simulink model "distributed_UIO_4nodes_directed"  (R2023a)
settings: Solver=VariableStepAuto  StartTime=0.0  StopTime=10  FixedStep=1e-6  RelTol=1e-6
values from neighbouring files (symbols this model uses):
  A = [-1   0    0   0   0   0 ... (first row only)    [init_simulink_DO.m]    (also in main.m)
  Adj = aij    [init_simulink_DO.m]
  gamma = 219.7065    [init_simulink_DO.m]    (also in main.m)
  H1 = [  1 0 0 2 0 0 ... (first row only)    [init_simulink_DO.m]    (also in main.m)
  H2 = [2 0 1 0 0 1]    [init_simulink_DO.m]    (also in main.m)
  H3 = [0 0 0 2 0 0]    [init_simulink_DO.m]    (also in main.m)
  H4 = [1 0 2 0 0 0 ... (first row only)    [init_simulink_DO.m]    (also in main.m)
  L1 = [0.1661 0.1661 ... (first row only)    [init_simulink_DO.m]    (also in main.m)
  L2 = [3.5770 ... (first row only)    [init_simulink_DO.m]    (also in main.m)
  L3 = [0 ... (first row only)    [init_simulink_DO.m]    (also in main.m)
  L4 = [-2.2551    0.3970 ... (first row only)    [init_simulink_DO.m]    (also in main.m)
  M1 = [0.0037    0       0   0       0   0 ... (first row only)    [init_simulink_DO.m]    (also in main.m)
  M2 = [0.0512     0.0879      -0.1315     -0.1416     -0.0429     0.0297 ... (first row only)    [init_simulink_DO.m]    (also in main.m)
  M3 = [1  0   0   0       0   0 ... (first row only)    [init_simulink_DO.m]    (also in main.m)
  M4 = [0.0390     0.0293      -0.0195     -0.1186     -0.1410     0.0409 ... (first row only)    [init_simulink_DO.m]    (also in main.m)
  x0 = [1, 3, -2, -3, -1, 2]'    [init_simulink_DO.m]
settings Model: Creator=gy116  LastModifiedBy=Quang Huy Nugyen
settings SolverCC: AlgebraicLoopSolver=LineSearch
settings DataIOCC: ReturnWorkspaceOutputs=off
settings DebuggingCC: UnconnectedInputMsg=warning  UnconnectedOutputMsg=warning  UnconnectedLineMsg=warning  ArithmeticOperatorsInVariantConditions=warning
settings ModelReferenceCC: EnableRefExpFcnMdlSchedulingChecks=on
settings SFSimCC: SimUseLocalCustomCode=off  CustomCodeUndefinedFunction=UseInterfaceOnly
settings RTWCC: RTWUseLocalCustomCode=off  DLArmComputeVersion=19.05
settings CodeAppCC: StateflowObjectComments=on

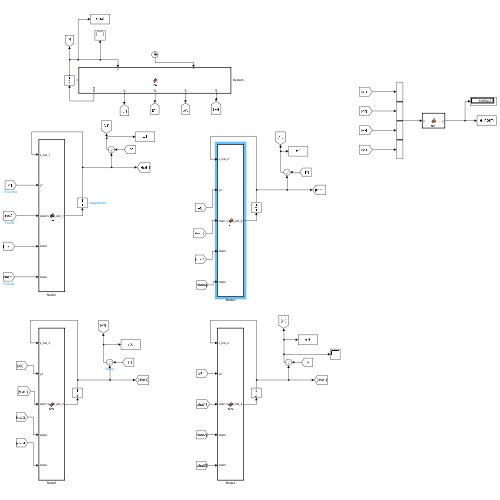
[thumbnail: Simulink's stored preview of the top-level diagram]
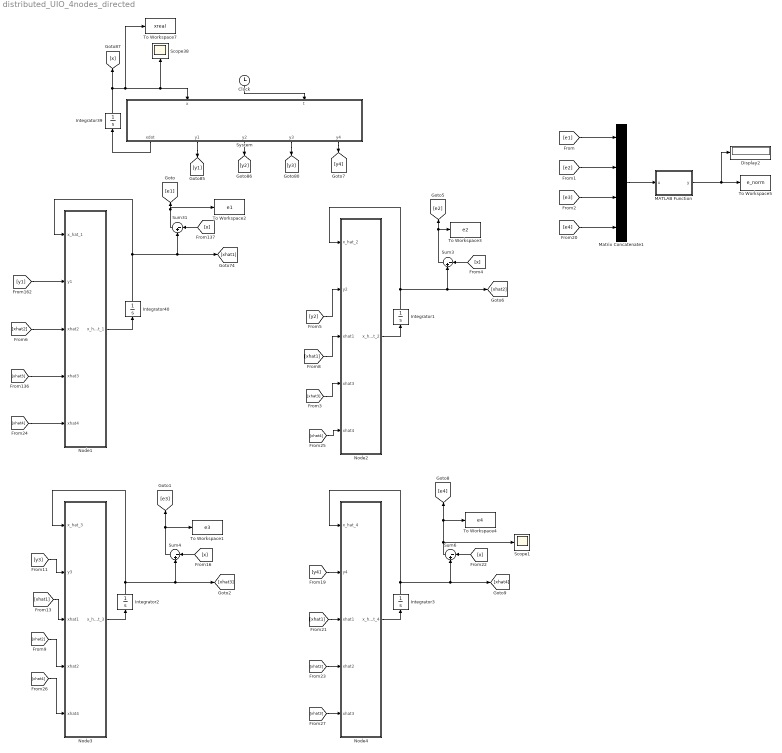
== system distributed_UIO_4nodes_directed ==
  Clock : Clock
  Display2 : Display
  Integrator{1..3,40} (4 alike) : Integrator  InitialCondition=0*x0
  Integrator39 : Integrator  InitialCondition=x0
  MATLAB Function : MATLAB Function  TreatAsAtomicUnit=on
  Matrix Concatenate1 : Concatenate  NumInputs=4  ConcatenateDimension=2
  Node1 : MATLAB Function  TreatAsAtomicUnit=on
  Node2 : MATLAB Function  TreatAsAtomicUnit=on
  Node3 : MATLAB Function  TreatAsAtomicUnit=on
  Node4 : MATLAB Function  TreatAsAtomicUnit=on
  Scope1 : Scope
  Scope38 : Scope
  Sum{3..4,6,31} (4 alike) : Sum  Inputs=|-+
  System : MATLAB Function  TreatAsAtomicUnit=on
  To Workspace1 : ToWorkspace  VariableName=e3  SaveFormat=Structure With Time  SampleTime=-1
  To Workspace2 : ToWorkspace  VariableName=e1  SaveFormat=Structure With Time  SampleTime=-1
  To Workspace3 : ToWorkspace  VariableName=e2  SaveFormat=Structure With Time  SampleTime=-1
  To Workspace4 : ToWorkspace  VariableName=e4  SaveFormat=Structure With Time  SampleTime=-1
  To Workspace5 : ToWorkspace  VariableName=e_norm  SaveFormat=Structure With Time  SampleTime=-1
  To Workspace7 : ToWorkspace  VariableName=xreal  SaveFormat=Structure With Time  SampleTime=-1
  wires:
  [e1] -> Matrix Concatenate1/1
  [e2] -> Matrix Concatenate1/2
  [e3] -> Matrix Concatenate1/3
  [e4] -> Matrix Concatenate1/4
  [x] -> Sum6/1
  [xhat1] -> Node3/3(xhat1)
  Sum6/1 -> Scope1/1, To Workspace4/1, [e4]
  Node1/1(x_hat_dot_1) -> Integrator40/1
  [y1] -> Node1/2(y1)
  Integrator2/1 -> Sum4/2, [xhat3], Node3/1(x_hat_3)
  Integrator40/1 -> Sum31/2, [xhat1], Node1/1(x_hat_1)
  Node4/1(x_hat_dot_4) -> Integrator3/1
  Integrator39/1 -> To Workspace7/1, System/1(x), Scope38/1, [x]
  Integrator1/1 -> Sum3/2, [xhat2], Node2/1(x_hat_2)
  [xhat4] -> Node2/5(xhat4)
  System/5(y4) -> [y4]
  System/2(y1) -> [y1]
  [y4] -> Node4/2(y4)
  [xhat2] -> Node4/4(xhat2)
  [xhat3] -> Node4/5(xhat3)
  Sum3/1 -> To Workspace3/1, [e2]
  System/1(xdot) -> Integrator39/1
  Clock/1 -> System/2(t)
  [xhat2] -> Node1/3(xhat2)
  System/4(y3) -> [y3]
  [x] -> Sum31/1
  [xhat4] -> Node3/5(xhat4)
  [y2] -> Node2/2(y2)
  [y3] -> Node3/2(y3)
  Sum31/1 -> To Workspace2/1, [e1]
  [xhat3] -> Node2/4(xhat3)
  [xhat2] -> Node3/4(xhat2)
  System/3(y2) -> [y2]
  [xhat3] -> Node1/4(xhat3)
  [x] -> Sum3/1
  Node2/1(x_hat_dot_2) -> Integrator1/1
  Node3/1(x_hat_dot_3) -> Integrator2/1
  [x] -> Sum4/1
  [xhat1] -> Node2/3(xhat1)
  Sum4/1 -> To Workspace1/1, [e3]
  Integrator3/1 -> Sum6/2, [xhat4], Node4/1(x_hat_4)
  [xhat1] -> Node4/3(xhat1)
  [xhat4] -> Node1/5(xhat4)
  Matrix Concatenate1/1 -> MATLAB Function/1(u)
  MATLAB Function/1(y) -> Display2/1, To Workspace5/1

== matlab function distributed_UIO_4nodes_directed/System ==
  data: x input; t input; A parameter; xdot output; y1 output; y2 output; y3 output; H2 parameter; H3 parameter; H1 parameter; H4 parameter; y4 output
function [xdot,y1,y2,y3,y4] = fcn(x,t,A,H2, H3, H1, H4)
xdot = A*x ;


y1 = H1*x;
y2 = H2*x;
y3 = H3*x;
y4 = H4*x;

== matlab function distributed_UIO_4nodes_directed/Node2 ==
  data: x_hat_2 input; y2 input; xhat1 input; xhat3 input; xhat4 input; x_hat_dot_2 output; L2 parameter; gamma parameter; Adj parameter; H2 parameter; A parameter; M2 parameter
function x_hat_dot_2   = fcn(x_hat_2,y2,xhat1,xhat3,xhat4,L2, gamma, Adj, H2, A, M2)

commu2 =  Adj(2,1)*(xhat1-x_hat_2) + Adj(2,3)*(xhat3-x_hat_2) + Adj(2,4)*(xhat4-x_hat_2);

x_hat_dot_2 = A*x_hat_2 + L2*(y2 - H2*x_hat_2) + gamma*M2*commu2;

== matlab function distributed_UIO_4nodes_directed/Node3 ==
  data: x_hat_3 input; y3 input; xhat1 input; xhat2 input; xhat4 input; M3 parameter; L3 parameter; Adj parameter; H3 parameter; x_hat_dot_3 output; A parameter; gamma parameter
function x_hat_dot_3   = fcn(x_hat_3,y3,xhat1,xhat2,xhat4,M3, L3, Adj, H3, A, gamma)

commu3 =  Adj(3,1)*(xhat1-x_hat_3) + Adj(3,2)*(xhat2-x_hat_3) +  Adj(3,4)*(xhat4-x_hat_3);

x_hat_dot_3 = A*x_hat_3 + L3*(y3 - H3*x_hat_3) + gamma*M3*commu3;

== matlab function distributed_UIO_4nodes_directed/Node4 ==
  data: x_hat_4 input; y4 input; xhat1 input; xhat2 input; xhat3 input; x_hat_dot_4 output; M4 parameter; L4 parameter; gamma parameter; Adj parameter; H4 parameter; A parameter
function x_hat_dot_4   = fcn(x_hat_4,y4,xhat1,xhat2,xhat3,M4, L4, gamma, Adj, H4, A)

commu4 =  Adj(4,1)*(xhat1 - x_hat_4) + Adj(4,2)*(xhat2 - x_hat_4) +  Adj(4,3)*(xhat3 - x_hat_4);

x_hat_dot_4 = A*x_hat_4 + L4*(y4 - H4*x_hat_4) + gamma*M4*commu4;

== matlab function distributed_UIO_4nodes_directed/MATLAB Function ==
  data: u input; y output
function y = fcn(u)

y = norm(u);

== matlab function distributed_UIO_4nodes_directed/Node1 ==
  data: x_hat_1 input; y1 input; xhat2 input; xhat3 input; xhat4 input; M1 parameter; L1 parameter; x_hat_dot_1 output; gamma parameter; Adj parameter; H1 parameter; A parameter
function x_hat_dot_1   = fcn(x_hat_1,y1,xhat2,xhat3,xhat4,M1, L1, gamma, Adj, H1, A)

commu1 =  Adj(1,2)*(xhat2-x_hat_1) + Adj(1,3)*(xhat3-x_hat_1) + Adj(1,4)*(xhat4-x_hat_1);

x_hat_dot_1 = A*x_hat_1 + L1*(y1 - H1*x_hat_1) + gamma*M1*commu1;
% x_hat_dot = A*x_hat_i + L_i*(y_i - H_i*x_hat_i) + gamma*M_i*commu;
